simulink model "MotorControlSimulation"  (R2026a)
settings: Solver=VariableStepAuto
libraries: mcbcontrolslib x1
settings Model: Creator=azmib  LastModifiedBy=azmib

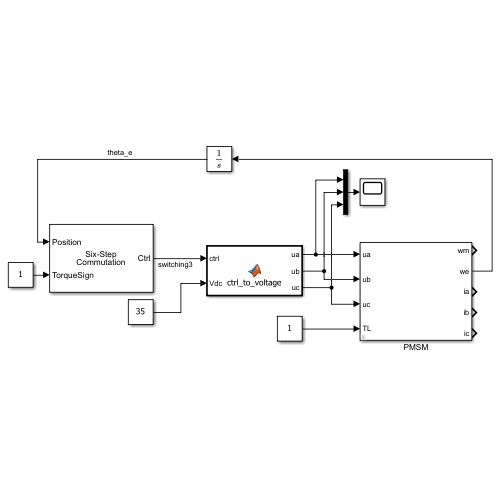
[thumbnail: Simulink's stored preview of the top-level diagram]
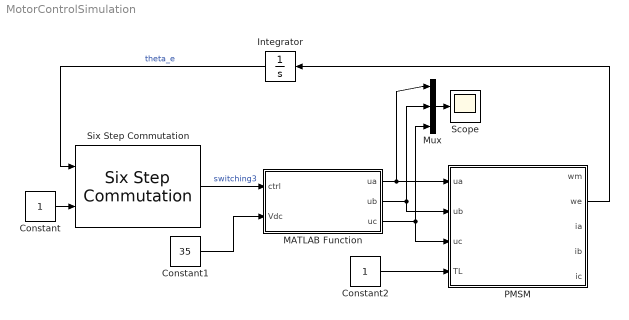
== system MotorControlSimulation ==
  Constant : Constant
  Constant1 : Constant  Value=35
  Constant2 : Constant
  Integrator : Integrator
  MATLAB Function : MATLAB Function  TreatAsAtomicUnit=on
  Mux : Mux  Inputs=3
  PMSM : Subsystem  mask(PMSM){Rs=0.045, Ls=18, psi_PM=0.018, p=14, J=2.5e-4, B=1e-5}
      mask prompts: Rs "Phase resistance [Rs]"; Ls "Direct- and  quadrature-axis inductances [Ls]"; psi_PM "Permanent magnet flux linkage [psi_PM]"; p "Pole pairs [p}"; J "Moment of inertia [J]"; B "viscous friction coefficient [B]"
      mask help: Mathematical model of a non-salient permanent magnet synchronous motor (PMSM).
  Scope : Scope
      settings: ActiveDisplayYMinimum=-7.7238272932970222  ActiveDisplayYMaximum=7.823564508493801
  Six Step Commutation : mcbcontrolslib/Six Step Commutation  InputType=Position  PositionUnit=Radians  CommutationMode=120 deg  SequencePos=[5,4,6,2,3,1]  EnableCustomSwitching=off  CommutationSeqPos=[0 0 1 0 0 1;0 1 1 0 0 0;0 1 0 0 1 0;0 0 0 1 1 0;1 0 0 1 0 0;1 0 0 0 0 1]  CommutationSeqNeg="[0  1  1  0  0  0;0  1  0  0  1  0;0  0  0  1  1  0;1  0  0  1  0  0;1  0  0  0  0  1;0  0  1  0  0  1;]"
      settings: LibrarySourceBlock=mcblib/Controls/Control Reference/Six Step Commutation
  wires:
  Integrator/1 -> Six Step Commutation/1  "theta_e"
  PMSM/2(we) -> Integrator/1
  Six Step Commutation/1 -> MATLAB Function/1(ctrl)  "switching3"
  Constant/1 -> Six Step Commutation/2
  Constant1/1 -> MATLAB Function/2(Vdc)
  MATLAB Function/1(ua) -> PMSM/1(ua), Mux/1
  MATLAB Function/2(ub) -> PMSM/2(ub), Mux/2
  MATLAB Function/3(uc) -> Mux/3, PMSM/3(uc)
  Constant2/1 -> PMSM/4(TL)
  Mux/1 -> Scope/1

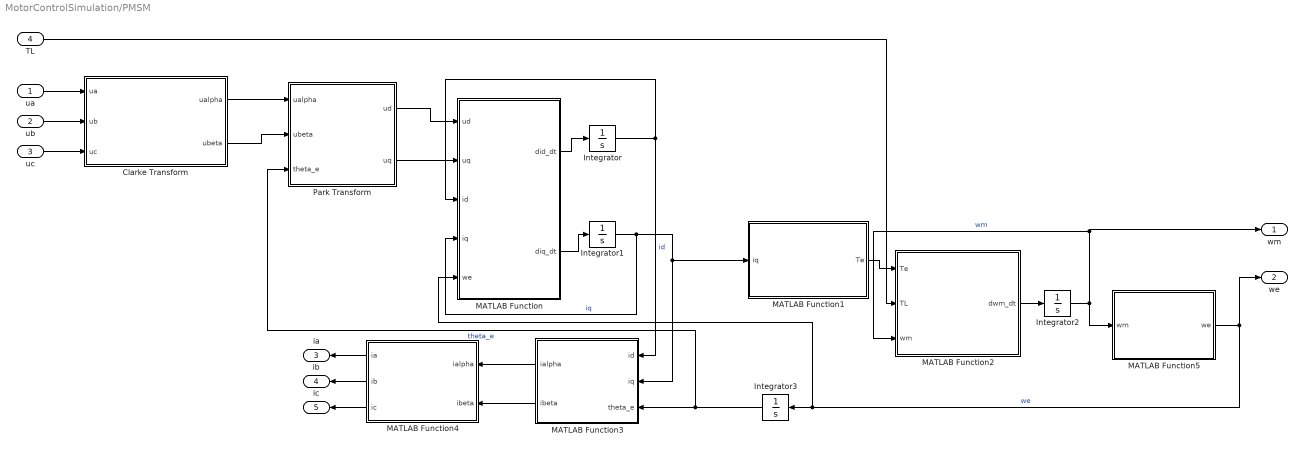
== system MotorControlSimulation/PMSM ==
  ua : Inport  Unit=V
  ub : Inport  Port=2  Unit=V
  uc : Inport  Port=3  Unit=V
  TL : Inport  Port=4
  Clarke Transform : MATLAB Function  TreatAsAtomicUnit=on
  Integrator{,1..3} (4 alike) : Integrator
  MATLAB Function : MATLAB Function  TreatAsAtomicUnit=on
  MATLAB Function1 : MATLAB Function  TreatAsAtomicUnit=on
  MATLAB Function2 : MATLAB Function  TreatAsAtomicUnit=on
  MATLAB Function3 : MATLAB Function  TreatAsAtomicUnit=on
  MATLAB Function4 : MATLAB Function  TreatAsAtomicUnit=on
  MATLAB Function5 : MATLAB Function  TreatAsAtomicUnit=on
  Park Transform : MATLAB Function  TreatAsAtomicUnit=on
  wm : Outport
  we : Outport  Port=2
  ia : Outport  Port=3
  ib : Outport  Port=4
  ic : Outport  Port=5
  wires:
  ua/1 -> Clarke Transform/1(ua)
  ub/1 -> Clarke Transform/2(ub)
  uc/1 -> Clarke Transform/3(uc)
  Clarke Transform/1(ualpha) -> Park Transform/1(ualpha)
  Clarke Transform/2(ubeta) -> Park Transform/2(ubeta)
  Park Transform/1(ud) -> MATLAB Function/1(ud)
  Park Transform/2(uq) -> MATLAB Function/2(uq)
  MATLAB Function/1(did_dt) -> Integrator/1
  MATLAB Function/2(diq_dt) -> Integrator1/1
  Integrator1/1 -> MATLAB Function3/2(iq), MATLAB Function1/1(iq), MATLAB Function/4(iq)  "iq"
  Integrator/1 -> MATLAB Function3/1(id), MATLAB Function/3(id)  "id"
  MATLAB Function1/1(Te) -> MATLAB Function2/1(Te)
  MATLAB Function2/1(dwm_dt) -> Integrator2/1
  Integrator2/1 -> MATLAB Function5/1(wm), wm/1, MATLAB Function2/3(wm)  "wm"
  MATLAB Function5/1(we) -> we/1, MATLAB Function/5(we), Integrator3/1  "we"
  Integrator3/1 -> MATLAB Function3/3(theta_e), Park Transform/3(theta_e)  "theta_e"
  MATLAB Function3/1(ialpha) -> MATLAB Function4/1(ialpha)
  MATLAB Function3/2(ibeta) -> MATLAB Function4/2(ibeta)
  MATLAB Function4/1(ia) -> ia/1
  MATLAB Function4/3(ic) -> ic/1
  MATLAB Function4/2(ib) -> ib/1
  TL/1 -> MATLAB Function2/2(TL)

== matlab function MotorControlSimulation/MATLAB Function ==
  data: ctrl input; ua output; Vdc input; ub output; uc output
function [ua, ub, uc] = ctrl_to_voltage(ctrl, Vdc)
% ctrl = [Aupper Alower Bupper Blower Cupper Clower]

ua = phase_voltage(ctrl(1), ctrl(2), Vdc);
ub = phase_voltage(ctrl(3), ctrl(4), Vdc);
uc = phase_voltage(ctrl(5), ctrl(6), Vdc);

end

function u = phase_voltage(upper, lower, Vdc)

if upper == 1 && lower == 0
    u = 0.5*Vdc;
elseif upper == 0 && lower == 1
    u = -0.5*Vdc;
else
    u = 0;
end

end

== matlab function MotorControlSimulation/PMSM/Park Transform ==
  data: ualpha input; ud output; ubeta input; theta_e input; uq output
function [ud, uq] = fcn_park(ualpha, ubeta, theta_e)
    c = cos(theta_e);
    s = sin(theta_e);
    T = [c,  s; ...
        -s,  c];
    uab = [ualpha; ubeta];
    udq = T * uab;
    ud = udq(1);
    uq = udq(2);
end

== matlab function MotorControlSimulation/PMSM/Clarke Transform ==
  data: ua input; ualpha output; ub input; uc input; ubeta output
function [ualpha, ubeta] = fcn_clarke(ua, ub, uc)
    T = (2/3) * [1, -0.5, -0.5; 0, sqrt(3)/2, -sqrt(3)/2];
    uabc = [ua; ub; uc];
    ualphabeta = T * uabc;
    ualpha = ualphabeta(1);
    ubeta  = ualphabeta(2);
end

== matlab function MotorControlSimulation/PMSM/MATLAB Function ==
  data: ud input; did_dt output; uq input; id input; iq input; we input; diq_dt output; Ls parameter; Rs parameter; psi_PM parameter
function [did_dt, diq_dt] = fcn_electrical_dyn(ud, uq, id, iq, we, Ls, Rs, psi_PM)
    % Avoid division by zero
    if Ls <= 0
        Ls = 1e-6;
    end
    
    did_dt = (ud - Rs*id + we*Ls*iq) / Ls;
    diq_dt = (uq - Rs*iq - we*(Ls*id + psi_PM)) / Ls;
end

== matlab function MotorControlSimulation/PMSM/MATLAB Function1 ==
  data: iq input; Te output; p parameter; psi_PM parameter
function Te = fcn_torque(iq, p, psi_PM)
    Te = 1.5 * p * psi_PM * iq;
end

== matlab function MotorControlSimulation/PMSM/MATLAB Function2 ==
  data: Te input; dwm_dt output; TL input; wm input; J parameter; B parameter
function dwm_dt = fcn_mechanical_dyn(Te, TL, wm, J, B)
    if J <= 0
        J = 1e-6;
    end
    dwm_dt = (Te - TL - B*wm) / J;
end

== matlab function MotorControlSimulation/PMSM/MATLAB Function3 ==
  data: id input; ialpha output; iq input; theta_e input; ibeta output
function [ialpha, ibeta] = fcn_inverseClarke(id, iq, theta_e)
    c = cos(theta_e);
    s = sin(theta_e);
    T = [c, -s; ...
         s,  c];
    idq = [id; iq];
    iab = T * idq;
    ialpha = iab(1);
    ibeta  = iab(2);
end

== matlab function MotorControlSimulation/PMSM/MATLAB Function4 ==
  data: ialpha input; ia output; ibeta input; ib output; ic output
function [ia, ib, ic] = fcn_inverseClarke(ialpha, ibeta)
    T = [1, 0; ...
        -0.5,  sqrt(3)/2; ...
        -0.5, -sqrt(3)/2];
    iab = [ialpha; ibeta];
    iabc = T * iab;
    ia = iabc(1);
    ib = iabc(2);
    ic = iabc(3);
end

== matlab function MotorControlSimulation/PMSM/MATLAB Function5 ==
  data: wm input; we output; p parameter
function we = fcn_wech2welec(wm, p)
    
    we = wm*p;
